simulink model "Communication1"  (R2020a)
settings: Solver=VariableStepAuto  StartTime=0.0  StopTime=0.6  RelTol=1e-3
settings Model: Creator=86188  LastModifiedBy=bzhan
settings DataIOCC: ReturnWorkspaceOutputs=off
settings DebuggingCC: ArithmeticOperatorsInVariantConditions=warning
settings SFSimCC: SimUseLocalCustomCode=off  CustomCodeUndefinedFunction=UseInterfaceOnly
settings RTWCC: RTWUseLocalCustomCode=off

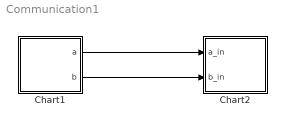
== system Communication1 ==
  Chart1 : Stateflow chart  TreatAsAtomicUnit=on
  Chart2 : Stateflow chart  TreatAsAtomicUnit=on
  wires:
  Chart1/2(b) -> Chart2/2(b_in)
  Chart1/1(a) -> Chart2/1(a_in)

== stateflow chart Communication1/Chart2 ==
  settings: updateMethod=DISCRETE  sampleTime=0.1
  state A1
    en: g("en_A1")
    du: f()
  (default) -> A1
  data: s function_input; a_in input; b_in input
  function f:
    | function f()
    |   fprintf("%.0f %.0f\n", a_in, b_in);
  function g(s):
    | function g(s)
    |   fprintf(s+"\n");

== stateflow chart Communication1/Chart1 ==
  settings: updateMethod=DISCRETE  sampleTime=0.1
  state A
    en:
    f("en_A")
  state B
    en:
    f("en_B")
  (default) -> A : {a=1;b=1;}
  A -> B : {a=a+1;}
  B -> A : {b=b+1;}
  data: s function_input; a output; b output
  function f(s):
    | function f(s)
    |   fprintf(s+"\n");
